simulink model "TPLIA_Input1"  (R2020b)
settings: Solver=VariableStepAuto  StartTime=0.0  StopTime=500  FixedStep=0.000001  MaxStep=1e-4  RelTol=1e-3  EnableMultiTasking=on
undefined symbols (not defined in the file): fdesignblkfcn, gcbh
libraries: dspfdesign x3, dspstat3 x3, dspsrcs4 x3, simulink x1, dsparch4 x1
settings Model: Creator=LYX  LastModifiedBy=LYX
settings DataIOCC: ReturnWorkspaceOutputs=off
settings OptimizationCC: DefaultUnderspecifiedDataType=single

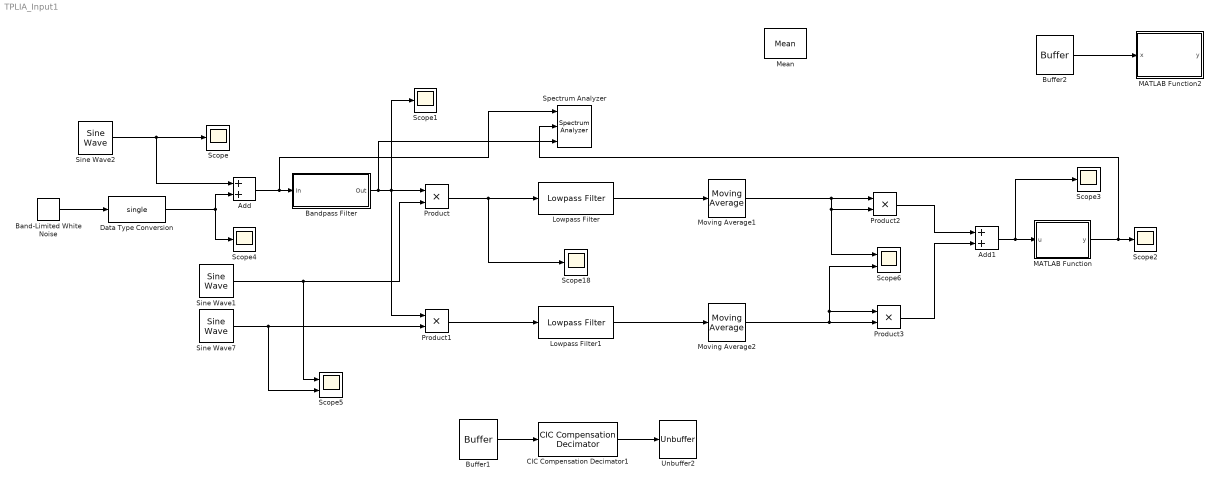
== system TPLIA_Input1 ==
  Add : Sum
  Add1 : Sum
  Band-Limited White Noise : simulink/Sources/Band-Limited White Noise  Cov=[0.0001*0.0001*1/240]  Ts=1/240  seed=[23341]
  Bandpass Filter : Subsystem  DialogController=fdesignblkfcn  InitFcn=fdesignblkfcn(gcbh, {'InitFcn'});  mask(Bandpass Filter){}
      mask help: Design a bandpass filter
      settings: CopyFcn=fdesignblkfcn(gcbh, {'CopyFcn'});
      mask Help: helpview(mapfilelocation('dsp'), 'dspbandpassfilter');
      mask Display: disp('Bandpass');
  Buffer1 : Buffer  N=4  OutputFrames=off
  Buffer2 : Buffer  N=240  V=180  OutputFrames=off
  CIC Compensation Decimator1 : dspfdesign/CIC Compensation Decimator  CICRateChangeFactor=6  CICNumSections=5  CICDifferentialDelay=1  DecimationFactor=4  DesignForMinimumOrder=on  FilterOrder=12  PassbandFrequency=0.3  StopbandFrequency=7.13  PassbandRipple=0.2  StopbandAttenuation=120  InheritSampleRate=off  SampleRate=960  SimulateUsing=Code generation  roundingMode=Floor  coeffsDataTypeStr=fixdt(1,16)
      settings: SourceProductBaseCode=DS
  Data Type Conversion : DataTypeConversion  OutDataTypeStr=single
  Lowpass Filter : dspfdesign/Lowpass Filter  FilterType=FIR  DesignForMinimumOrder=on  FilterOrder=50  PassbandFrequency=0.3  StopbandFrequency=1.5  PassbandRipple=2  StopbandAttenuation=90  InheritSampleRate=on  SampleRate=44100  SimulateUsing=Interpreted execution  roundingMode=Floor  coeffsDataTypeStr=fixdt(1,16)
  Lowpass Filter1 : dspfdesign/Lowpass Filter  FilterType=IIR  DesignForMinimumOrder=on  FilterOrder=50  PassbandFrequency=0.3  StopbandFrequency=1.5  PassbandRipple=2  StopbandAttenuation=90  InheritSampleRate=on  SampleRate=44100  SimulateUsing=Interpreted execution  roundingMode=Floor  coeffsDataTypeStr=fixdt(1,16)
  MATLAB Function : MATLAB Function  TreatAsAtomicUnit=on
  MATLAB Function2 : MATLAB Function  TreatAsAtomicUnit=on
  Mean : dspstat3/Mean  run=on  InputProcessing=Columns as channels (frame based)  reset_popup=None  directionMode=Each column  dimension=1  roiEnable=off  roiType=Rectangles  roiPortion=Entire ROI  roiOutput=Individual statistics for each ROI  roiFlag=off  roundingMode=Floor  overflowMode=off  outputDataTypeStr=Inherit: Same as accumulator  outputMin=[]  outputMax=[]  outputLastDataTypeStr=Inherit: Same as accumulator
  Moving Average1 : dspstat3/Moving Average  Method=Sliding window  ForgettingFactorPort=off  SpecifyWindowLength=on  WindowLength=180  ForgettingFactor=0.9  SimulateUsing=Code generation
  Moving Average2 : dspstat3/Moving Average  Method=Sliding window  ForgettingFactorPort=off  SpecifyWindowLength=on  WindowLength=180  ForgettingFactor=0.9  SimulateUsing=Code generation
  Product{,1..3} (4 alike) : Product
  Scope{,1..4,18} (6 alike) : Scope
  Scope5 : Scope  NumInputPorts=2
  Scope6 : Scope  NumInputPorts=2
  Sine Wave1 : dspsrcs4/Sine Wave  Amplitude=1  Frequency=20  Phase=0  SampleMode=Discrete  OutComplex=Real  CompMethod=Table lookup  TableSize=Speed  SampleTime=1/240  SamplesPerFrame=1  ResetState=Restart at time zero  OutputFrames=off  dataType=single  wordLen=16  udDataType=sfix(16)  fracBitsMode=Best precision  numFracBits=15  OutDataTypeStr=single  LastOutDataTypeStr=single
  Sine Wave2 : dspsrcs4/Sine Wave  Amplitude=0.001  Frequency=20  Phase=0  SampleMode=Discrete  OutComplex=Real  CompMethod=Trigonometric fcn  TableSize=Speed  SampleTime=1/240  SamplesPerFrame=1  ResetState=Restart at time zero  OutputFrames=off  dataType=single  wordLen=16  udDataType=sfix(16)  fracBitsMode=Best precision  numFracBits=15  OutDataTypeStr=single  LastOutDataTypeStr=single
  Sine Wave7 : dspsrcs4/Sine Wave  Amplitude=1  Frequency=20  Phase=pi/2  SampleMode=Discrete  OutComplex=Real  CompMethod=Table lookup  TableSize=Speed  SampleTime=1/240  SamplesPerFrame=1  ResetState=Restart at time zero  OutputFrames=off  dataType=single  wordLen=16  udDataType=sfix(16)  fracBitsMode=Best precision  numFracBits=15  OutDataTypeStr=single  LastOutDataTypeStr=single
  Spectrum Analyzer : SpectrumAnalyzer  NumInputPorts=3
  Unbuffer2 : Unbuffer
  wires:
  Sine Wave2/1 -> Add/1, Scope/1
  Sine Wave1/1 -> Scope5/1, Product/2
  Sine Wave7/1 -> Scope5/2, Product1/2
  Product2/1 -> Add1/1
  Product3/1 -> Add1/2
  Add1/1 -> Scope3/1, MATLAB Function/1(u)
  Product/1 -> Scope18/1, Lowpass Filter/1
  MATLAB Function/1(y) -> Spectrum Analyzer/2, Scope2/1
  CIC Compensation Decimator1/1 -> Unbuffer2/1
  Buffer1/1 -> CIC Compensation Decimator1/1
  Product1/1 -> Lowpass Filter1/1
  Data Type Conversion/1 -> Add/2, Scope4/1
  Buffer2/1 -> MATLAB Function2/1(x)
  Lowpass Filter/1 -> Moving Average1/1
  Moving Average1/1 -> Scope6/1, Product2/2, Product2/1
  Lowpass Filter1/1 -> Moving Average2/1
  Moving Average2/1 -> Product3/2, Scope6/2, Product3/1
  Add/1 -> Spectrum Analyzer/1, Bandpass Filter/1(In)
  Bandpass Filter/1(Out) -> Spectrum Analyzer/3, Product1/1, Product/1, Scope1/1
  Band-Limited White Noise/1 -> Data Type Conversion/1

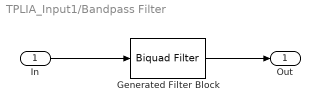
== system TPLIA_Input1/Bandpass Filter ==
  In : Inport
  Generated Filter Block : dsparch4/Biquad Filter  Tag=BlockMethodSubSystem  FilterSource=Dialog parameters  CoeffSource=Specify via dialog  FilterObject=BQF  IIRFiltStruct=Direct form II  BiQuadCoeffs=[0.0424025583404784023 0 -0.0424025583404784023 1 -1.72292226685437 0.96636319141191318;0.0251492877545773132 0 -0.0251492877545773132 1 -1.68057526496149867 0.963931146758460144;0.0285408999919945644 0 -0.0285408999919945644 1 -1.69665850844685795 0.94998076546523802;0.00828982610409956071 0 -0.00828982610409956071 1 -1.68063828580044694 0.948671315820520888;0.0548085450020374884 0 -0.0548085450020374884 1 -1.75177422420760864 0.992678427059907054;0.023906891706697686 0 -0.023906891706697686 1 -1.69774198836369106 0.99196798210601167;0.045529638637857299 0 -0.045529638637857299 1 -1.70896885669192189 0.956546379989341111;0.0272433095891107188 0 -0.0272433095891107188 1 -1.67839927713371528 0.954331122468260906;0.0137958410564951502 0 -0.0137958410564951502 1 -1.68693732130312912 0.947239933893518793;0.0502686436120278746 0 -0.0502686436120278746 1 -1.73752405857869174 0.978692728532177258;1.0364697615169034 0 -1.0364697615169034 1 -1.68716105651849047 0.976813679097303766]  ScaleValues=[0.0162035224683577984;1;1;1;1;1;1;1;1;1;1;1]  IC=0  ICnum=0  ICden=0  a0Flag=Warning  optimizeScaleValues=off  ScaleValueMode=Specify via input port (g)  InputProcessing=Columns as channels (frame based)  roundingMode=Floor  overflowMode=off  scaleValueFracLength=14  denProdOutputFracLength=30  denAccumFracLength=30  secondMemoryFracLength=15
  Out : Outport  VectorParamsAs1DForOutWhenUnconnected=off
  wires:
  In/1 -> Generated Filter Block/1
  Generated Filter Block/1 -> Out/1

== matlab function TPLIA_Input1/MATLAB Function2 ==
  data: x input; y output
function y = average(x)
    y=mean(x);
end

== matlab function TPLIA_Input1/MATLAB Function ==
  data: u input; y output
function y = fcn(u)

y = 2 * sqrt(u);
